simulink model "untitled"  (Simulink 8.1)
settings: Solver=ode45  SolverMode=SingleTasking  StartTime=0.0  StopTime=50  RelTol=1e-3
libraries: fuzblock x3, simulink x1
settings Model: Creator=Abu Fayez  LastModifiedBy=Abu Fayez  CovMetricSettings=dwe  CovHtmlReporting=off  covSaveCumulativeToWorkspaceVar=off  CovSaveSingleToWorkspaceVar=off  CovExternalEMLEnable=on
settings DataIOCC: LimitDataPoints=off  SaveFormat=StructureWithTime  SignalLoggingSaveFormat=Dataset
settings OptimizationCC: ExpressionDepthLimit=128
settings DebuggingCC: UnderspecifiedInitializationDetection=Simplified  MergeDetectMultiDrivingBlocksExec=error  SolverPrmCheckMsg=none  FcnCallInpInsideContextMsg=EnableAllAsError  FrameProcessingCompatibilityMsg=error  StateNameClashWarn=none  SFUnexpectedBacktrackingDiag=error  SFNoUnconditionalDefaultTransitionDiag=error
settings HardwareCC: ProdBitPerPointer=64  ProdLargestAtomicFloat=Float  ProdIntDivRoundTo=Zero  ProdEndianess=LittleEndian  ProdHWDeviceType=Specified
settings ModelReferenceCC: PropagateSignalLabelsOutOfModel=on
settings GRTTargetCC: CodeReplacementLibrary=C99 (ISO)  GeneratePreprocessorConditionals=Use local settings  CombineOutputUpdateFcns=on  GRTInterface=off

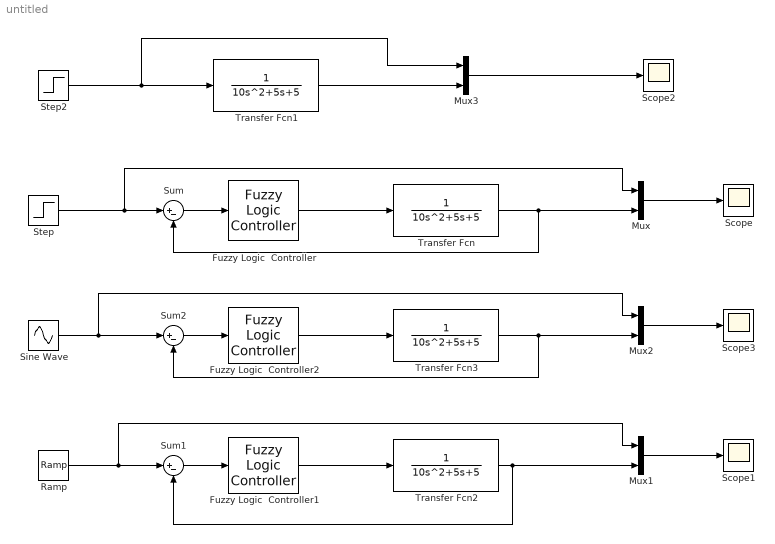
== system untitled ==
  Fuzzy Logic  Controller : fuzblock/Fuzzy Logic  Controller  FIS=Untitled4
  Fuzzy Logic  Controller1 : fuzblock/Fuzzy Logic  Controller  FIS=Untitled4
  Fuzzy Logic  Controller2 : fuzblock/Fuzzy Logic  Controller  FIS=Untitled4
  Mux{,1..3} (4 alike) : Mux  Inputs=2
  Ramp : simulink/Sources/Ramp  slope=.1  start=0  X0=0
  Scope{,1..3} (4 alike) : Scope
      Scope settings: TimeRange=auto  MaxDataPoints=5000  SaveToWorkspace=off  YMin=-0.71139  YMax=6.40252  SampleTime=-1
      Scope1 settings: TimeRange=auto  MaxDataPoints=5000  SaveToWorkspace=off  SaveName=ScopeData2  YMin=-0.57586  YMax=5.18273  SampleTime=-1
      Scope2 settings: TimeRange=auto  MaxDataPoints=5000  SaveToWorkspace=off  SaveName=ScopeData2  YMin=-6.25  YMax=56.25  SampleTime=-1
      Scope3 settings: TimeRange=auto  MaxDataPoints=5000  SaveToWorkspace=off  SaveName=ScopeData3  YMin=-8.84526  YMax=8.87786  SampleTime=-1
  Sine Wave : Sin  Amplitude=5  SampleTime=0
  Step : Step  After=5  SampleTime=0
  Step2 : Step  After=50  SampleTime=0
  Sum : Sum  Inputs=|+-
  Sum1 : Sum  Inputs=|+-
  Sum2 : Sum  Inputs=|+-
  Transfer Fcn{,1..3} (4 alike) : TransferFcn  Denominator=[10 5 5]
  wires:
  Fuzzy Logic  Controller/1 -> Transfer Fcn/1
  Step2/1 -> Mux3/1, Transfer Fcn1/1
  Mux3/1 -> Scope2/1
  Transfer Fcn1/1 -> Mux3/2
  Transfer Fcn/1 -> Sum/2, Mux/2
  Sum/1 -> Fuzzy Logic  Controller/1
  Mux/1 -> Scope/1
  Step/1 -> Mux/1, Sum/1
  Fuzzy Logic  Controller1/1 -> Transfer Fcn2/1
  Transfer Fcn2/1 -> Mux1/2, Sum1/2
  Ramp/1 -> Sum1/1, Mux1/1
  Mux1/1 -> Scope1/1
  Sum1/1 -> Fuzzy Logic  Controller1/1
  Sum2/1 -> Fuzzy Logic  Controller2/1
  Mux2/1 -> Scope3/1
  Transfer Fcn3/1 -> Mux2/2, Sum2/2
  Fuzzy Logic  Controller2/1 -> Transfer Fcn3/1
  Sine Wave/1 -> Sum2/1, Mux2/1
